simulink model "Virtual_Engine_Airpath_Model"  (R2016b)
settings: Solver=FixedStepDiscrete  StartTime=0.0  StopTime=inf  FixedStep=VirtEngAirPathMdl.tiSimnTiStep_C.Value  RelTol=1e-3  EnableMultiTasking=on
InitFcn:
  | % Call parameters initialization function
  | % run optiTruck_init_sim.m;
StopFcn:
  | %optiTruck_post_sim;
  | %optiTruck_plot_sim;
settings Model: Creator=engin  LastModifiedBy=bunver
settings DataIOCC: SaveFormat=StructureWithTime  SaveOutput=off  DSMLogging=off  VisualizeSimOutput=off  SaveTime=off  SignalLoggingName=Results
settings OptimizationCC: BlockReduction=off  ConditionallyExecuteInputs=off  LifeSpan=inf
settings DebuggingCC: AllowSymbolicDim=off  SFUnexpectedBacktrackingDiag=warning  SFNoUnconditionalDefaultTransitionDiag=warning  SFExecutionAtInitializationDiag=none
settings ModelReferenceCC: ModelReferenceNumInstancesAllowed=Single  PropagateSignalLabelsOutOfModel=off
settings GRTTargetCC: TargetLangStandard=C89/C90 (ANSI)
settings ConfigComp: CovMetricSettings=dw  CovHtmlReporting=on  CovSaveCumulativeToWorkspaceVar=on  CovSaveSingleToWorkspaceVar=on  CovExternalEMLEnable=off

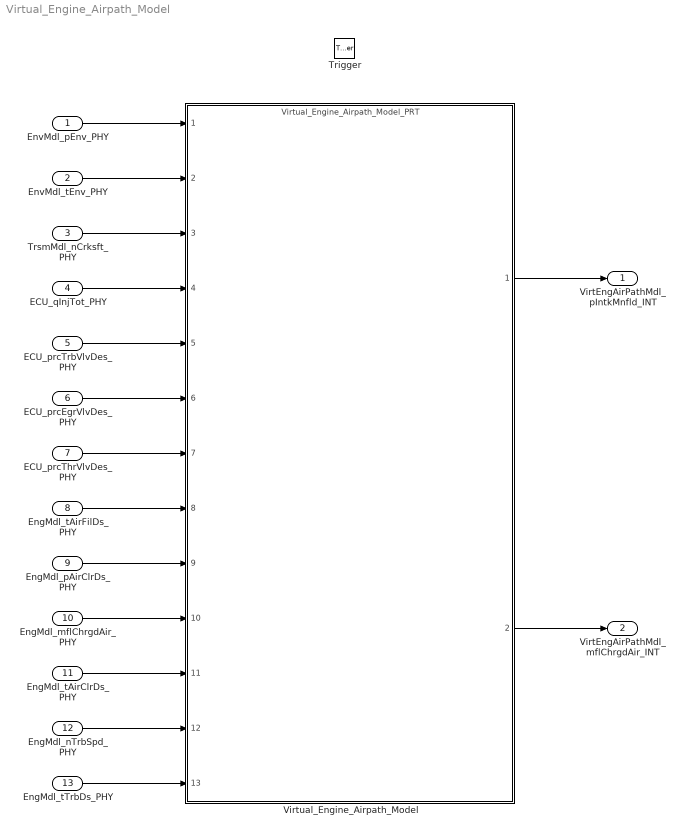
== system Virtual_Engine_Airpath_Model ==
  EnvMdl_pEnv_PHY : Inport
  EnvMdl_tEnv_PHY : Inport  Port=2
  TrsmMdl_nCrksft_PHY : Inport  Port=3
  ECU_qInjTot_PHY : Inport  Port=4
  ECU_prcTrbVlvDes_PHY : Inport  Port=5
  ECU_prcEgrVlvDes_PHY : Inport  Port=6
  ECU_prcThrVlvDes_PHY : Inport  Port=7
  EngMdl_tAirFilDs_PHY : Inport  Port=8
  EngMdl_pAirClrDs_PHY : Inport  Port=9
  EngMdl_mflChrgdAir_PHY : Inport  Port=10
  EngMdl_tAirClrDs_PHY : Inport  Port=11
  EngMdl_nTrbSpd_PHY : Inport  Port=12
  EngMdl_tTrbDs_PHY : Inport  Port=13
  Trigger : TriggerPort  TriggerType=function-call  VariantControl=Variant  PortDimensions=1
  Virtual_Engine_Airpath_Model : ModelReference  ModelNameDialog=Virtual_Engine_Airpath_Model_PRT.slx  ModelReferenceVersion=1.191
  VirtEngAirPathMdl_pIntkMnfld_INT : Outport
  VirtEngAirPathMdl_mflChrgdAir_INT : Outport  Port=2
  wires:
  EnvMdl_pEnv_PHY/1 -> Virtual_Engine_Airpath_Model/1
  EnvMdl_tEnv_PHY/1 -> Virtual_Engine_Airpath_Model/2
  TrsmMdl_nCrksft_PHY/1 -> Virtual_Engine_Airpath_Model/3
  ECU_qInjTot_PHY/1 -> Virtual_Engine_Airpath_Model/4
  ECU_prcTrbVlvDes_PHY/1 -> Virtual_Engine_Airpath_Model/5
  ECU_prcEgrVlvDes_PHY/1 -> Virtual_Engine_Airpath_Model/6
  ECU_prcThrVlvDes_PHY/1 -> Virtual_Engine_Airpath_Model/7
  EngMdl_tAirFilDs_PHY/1 -> Virtual_Engine_Airpath_Model/8
  EngMdl_pAirClrDs_PHY/1 -> Virtual_Engine_Airpath_Model/9
  EngMdl_mflChrgdAir_PHY/1 -> Virtual_Engine_Airpath_Model/10
  EngMdl_tAirClrDs_PHY/1 -> Virtual_Engine_Airpath_Model/11
  EngMdl_nTrbSpd_PHY/1 -> Virtual_Engine_Airpath_Model/12
  EngMdl_tTrbDs_PHY/1 -> Virtual_Engine_Airpath_Model/13
  Virtual_Engine_Airpath_Model/1 -> VirtEngAirPathMdl_pIntkMnfld_INT/1
  Virtual_Engine_Airpath_Model/2 -> VirtEngAirPathMdl_mflChrgdAir_INT/1
